simulink subsystem "UDP_MCU"  (R2019b)
settings: Solver=VariableStepAuto  StartTime=0.0  StopTime=10.0  RelTol=1e-3
libraries: xpcrtudplib x3, xpcutilitieslib x2
settings Model: Creator=toons  LastModifiedBy=toons

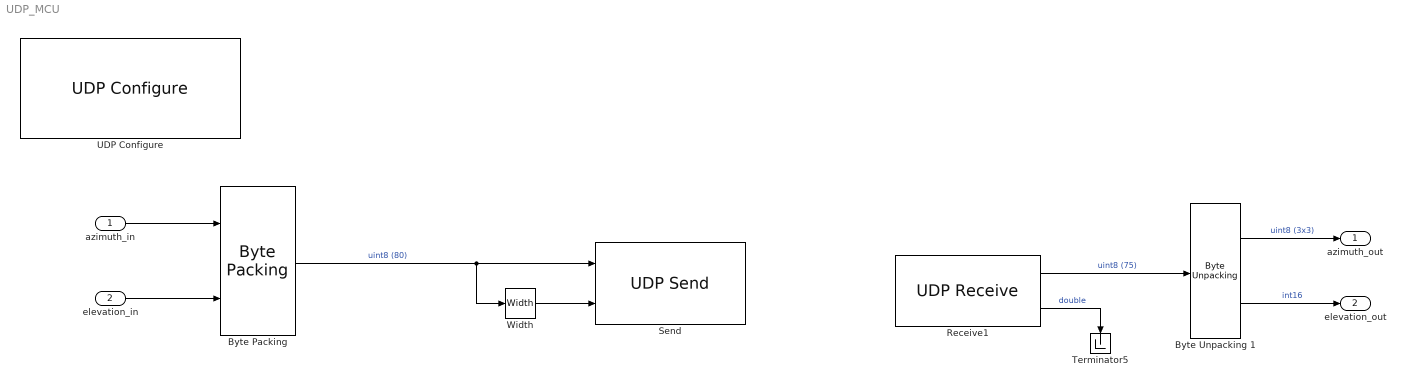
== system UDP_MCU ==
  azimuth_in : Inport
  elevation_in : Inport  Port=2
  "Byte Packing " : xpcutilitieslib/Byte Packing   MaskPackedDataType=uint8  MaskUnpackedDataTypes={'double', 'double'}  MaskAlignment=1
  Byte Unpacking 1 : xpcutilitieslib/Byte Unpacking   MaskUnpackedDataTypes={'double','double'}  MaskUnpackedDataSizes={[1],[1]}  MaskAlignment=1
      settings: SourceProductName=Simulink Real-Time  SourceProductBaseCode=XP
  Receive1 : xpcrtudplib/UDP Receive  Priority=4  ipAddressVal=Use host-target connection  localPort=25000  rcvWidth=16  rcvFmAny=off  fmAddress=127.0.0.1  rcvMulticast=off  multicastAddress={}  maxUDPQueue=8  sampleTime=0.01
      settings: SourceProductName=Simulink Real-Time
  Send : xpcrtudplib/UDP Send  Priority=3  ipAddressVal=Use host-target connection  localPort=-1  toAddress=127.0.0.1  toPort=25000  sampleTime=0.01
      settings: SourceProductName=Simulink Real-Time  SourceProductBaseCode=XP
  Terminator5 : Terminator
  UDP Configure : xpcrtudplib/UDP Configure  Priority=-1  IpAddress=127.0.0.1  SubnetMask=255.255.255.0  Gateway=0.0.0.0  PciBus=5  PciSlot=1  PciFunction=0  ID=1  tune=0  disable=off  enableMulticast=off  MulticastIpAddress={}  MulticastMask={}
      settings: SourceProductName=Simulink Real-Time  SourceProductBaseCode=XP
  Width : Width
  azimuth_out : Outport
  elevation_out : Outport  Port=2
  wires:
  Receive1/1 -> Byte Unpacking 1/1  "uint8 (75)"
  Receive1/2 -> Terminator5/1  "double"
  "Byte Packing "/1 -> Send/1, Width/1  "uint8 (80)"
  Width/1 -> Send/2
  azimuth_in/1 -> "Byte Packing "/1
  elevation_in/1 -> "Byte Packing "/2
  Byte Unpacking 1/1 -> azimuth_out/1  "uint8 (3x3)"
  Byte Unpacking 1/2 -> elevation_out/1  "int16"
